simulink subsystem "IdealVoltageSource"  (R2025b)
settings: Solver=VariableStepAuto  StartTime=0.0  StopTime=10.0  RelTol=1e-3
undefined symbols (not defined in the file): PlntBattIdealSoc, PlntBattIdealVolt, PlntBattNumCellSer, PlntBattTempInitDegC
settings Model: ModifiedByFormat=The MathWorks, Inc.  Creator=The MathWorks, Inc.  LastModifiedBy=The MathWorks, Inc.
settings SolverCC: MaxZcPerStep=1.0
settings OptimizationCC: ReuseModelBlockBuffer=off
settings DebuggingCC: UnconnectedInputMsg=warning  UnconnectedOutputMsg=warning  UnconnectedLineMsg=warning
settings ModelReferenceCC: EnableRefExpFcnMdlSchedulingChecks=on
settings RTWCC: GPUComputeCapability=3.5  DLArmComputeVersion=19.05

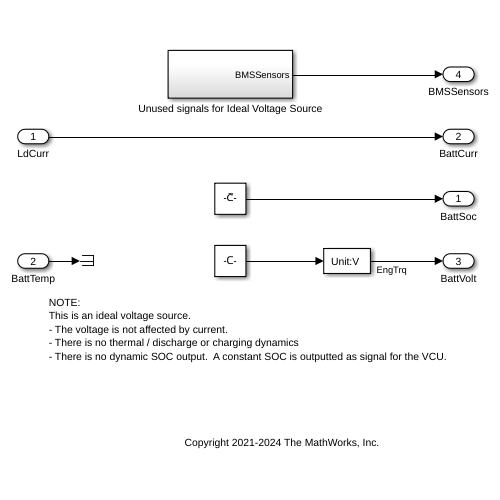
[thumbnail: Simulink's stored preview of the top-level diagram]
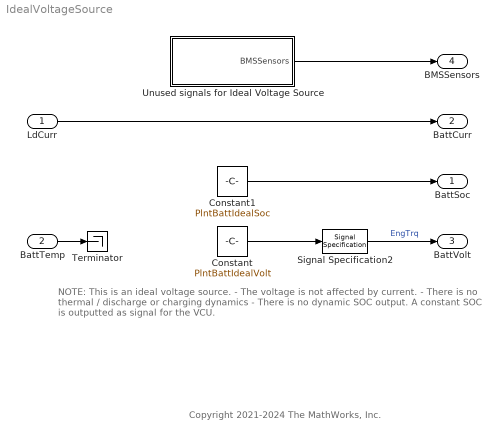
== system IdealVoltageSource ==
  note: NOTE:
      | This is an ideal voltage source.
      | - The voltage is not affected by current.
      | - There is no thermal / discharge or charging dynamics
      | - There is no dynamic SOC output.  A constant SOC is outputted as signal for the VCU.
  note: Copyright 2021-2024 The MathWorks, Inc.
  LdCurr : Inport
  BattTemp : Inport  Port=2
  Constant : Constant  Value=PlntBattIdealVolt  SampleTime=-1
  Constant1 : Constant  Value=PlntBattIdealSoc  SampleTime=-1
  Signal Specification2 : SignalSpecification  Unit=V
  Terminator : Terminator
  Unused signals for Ideal Voltage Source : Subsystem
  BattSoc : Outport  VectorParamsAs1DForOutWhenUnconnected=off
  BattCurr : Outport  Port=2  VectorParamsAs1DForOutWhenUnconnected=off
  BattVolt : Outport  Port=3  VectorParamsAs1DForOutWhenUnconnected=off
  BMSSensors : Outport  Port=4  VectorParamsAs1DForOutWhenUnconnected=off
  wires:
  Constant1/1 -> BattSoc/1
  LdCurr/1 -> BattCurr/1
  BattTemp/1 -> Terminator/1
  Constant/1 -> Signal Specification2/1
  Signal Specification2/1 -> BattVolt/1  "EngTrq"
  Unused signals for Ideal Voltage Source/1(BMSSensors) -> BMSSensors/1

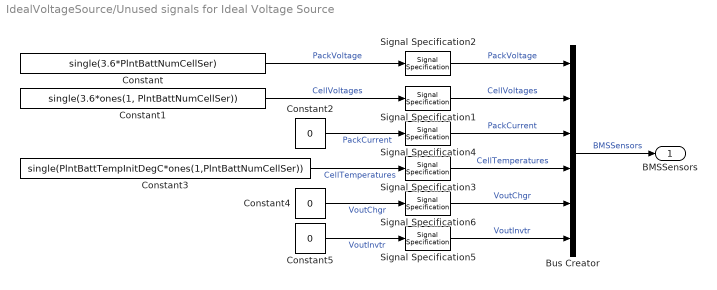
== system IdealVoltageSource/Unused signals for Ideal Voltage Source ==
  Bus Creator : BusCreator  Inputs=6
  Constant : Constant  Value=single(3.6*PlntBattNumCellSer)  SampleTime=-1
  Constant1 : Constant  Value=single(3.6*ones(1, PlntBattNumCellSer))  SampleTime=-1
  Constant2 : Constant  Value=0  OutDataTypeStr=single  SampleTime=-1
  Constant3 : Constant  Value=single(PlntBattTempInitDegC*ones(1,PlntBattNumCellSer))  SampleTime=-1
  Constant4 : Constant  Value=0  OutDataTypeStr=single  SampleTime=-1
  Constant5 : Constant  Value=0  OutDataTypeStr=single  SampleTime=-1
  Signal Specification{1..2,5..6} (4 alike) : SignalSpecification  Unit=V
  Signal Specification3 : SignalSpecification  Unit=°C
  Signal Specification4 : SignalSpecification  Unit=A
  BMSSensors : Outport
  wires:
  Constant/1 -> Signal Specification2/1  "PackVoltage"
  Signal Specification2/1 -> Bus Creator/1  "PackVoltage"
  Signal Specification1/1 -> Bus Creator/2  "CellVoltages"
  Constant1/1 -> Signal Specification1/1  "CellVoltages"
  Constant3/1 -> Signal Specification3/1  "CellTemperatures"
  Constant2/1 -> Signal Specification4/1  "PackCurrent"
  Constant4/1 -> Signal Specification6/1  "VoutChgr"
  Constant5/1 -> Signal Specification5/1  "VoutInvtr"
  Signal Specification4/1 -> Bus Creator/3  "PackCurrent"
  Signal Specification3/1 -> Bus Creator/4  "CellTemperatures"
  Signal Specification6/1 -> Bus Creator/5  "VoutChgr"
  Signal Specification5/1 -> Bus Creator/6  "VoutInvtr"
  Bus Creator/1 -> BMSSensors/1  "BMSSensors"
